simulink model "rotation_controllers_test"  (Simulink 8.8)
settings: Solver=ode4  StartTime=0.0  StopTime=10.0  FixedStep=1e-4  RelTol=1e-3  EnableMultiTasking=on
values from neighbouring files (symbols this model uses):
  g = [0;0;-9.81]    [rotation_controllers_test_start.m]
  I_B_C = inertiavector2matrix([4, 8, 15,-1,-2,-0.5])    [rotation_controllers_test_start.m]
  m = 1.5    [rotation_controllers_test_start.m]
libraries: lib_cartesian_controllers x2, rigid_body_dynamics x2, transformations_lib x2
settings Model: SuppressorTable=22 serialization::archive 11 0 3 0 0 0 11 0  Creator=schappler  LastModifiedBy=schappler
settings DataIOCC: LimitDataPoints=off  SaveFormat=StructureWithTime  SignalLoggingSaveFormat=Dataset
settings DebuggingCC: UnderspecifiedInitializationDetection=Simplified  MergeDetectMultiDrivingBlocksExec=error  FcnCallInpInsideContextMsg=error  StateNameClashWarn=none
settings GRTTargetCC: CombineOutputUpdateFcns=on  GRTInterface=off

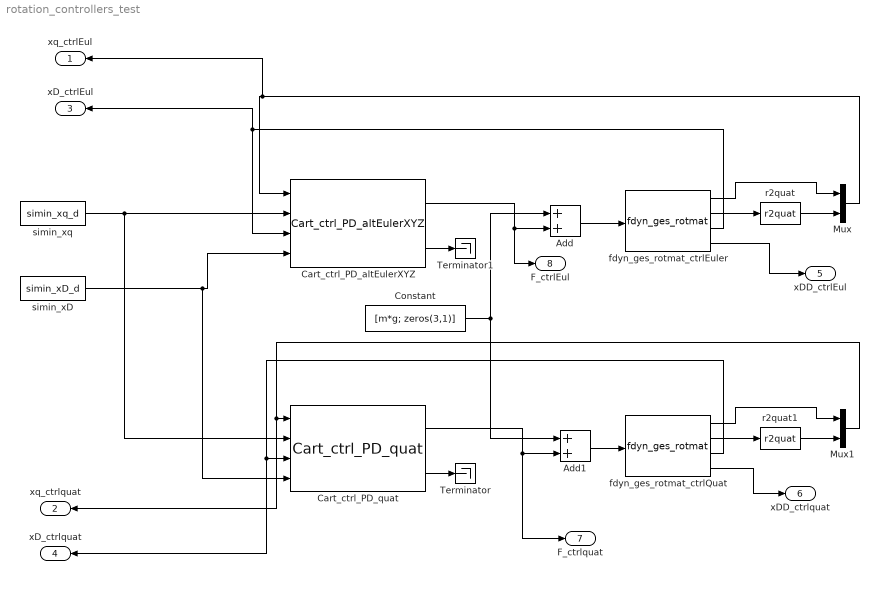
== system rotation_controllers_test ==
  Add : Sum
  Add1 : Sum
  Cart_ctrl_PD_altEulerXYZ : lib_cartesian_controllers/Cart_ctrl_PD_altEulerXYZ  k_P_p=k_P_p_C1  k_P_r=k_P_r_C1  k_D_p=k_D_p_C1  k_D_r=k_D_r_C1
  Cart_ctrl_PD_quat : lib_cartesian_controllers/Cart_ctrl_PD_quat  k_P_p=k_P_p_C2  k_P_r=k_P_r_C2  k_D_p=k_D_p_C2  k_D_r=k_D_r_C2
  Constant : Constant  Value=[m*g; zeros(3,1)]
  Mux : Mux  Inputs=[3 4]
  Mux1 : Mux  Inputs=[3 4]
  Terminator : Terminator
  Terminator1 : Terminator
  fdyn_ges_rotmat_ctrlEuler : rigid_body_dynamics/fdyn_ges_rotmat  I=I_B_C  m=m  r0=r0  rD0=rD0  R_t0=R_W_B_t0  omega0_t0=omega0_t0  r_B_B_C=r_B_B_C
  fdyn_ges_rotmat_ctrlQuat : rigid_body_dynamics/fdyn_ges_rotmat  I=I_B_C  m=m  r0=r0  rD0=rD0  R_t0=R_W_B_t0  omega0_t0=omega0_t0  r_B_B_C=r_B_B_C
  r2quat : transformations_lib/r2quat
  r2quat1 : transformations_lib/r2quat
  simin_xD : FromWorkspace  VariableName=simin_xD_d  SampleTime=0
  simin_xq : FromWorkspace  VariableName=simin_xq_d  SampleTime=0
  xq_ctrlEul : Outport
  xq_ctrlquat : Outport  Port=2
  xD_ctrlEul : Outport  Port=3
  xD_ctrlquat : Outport  Port=4
  xDD_ctrlEul : Outport  Port=5
  xDD_ctrlquat : Outport  Port=6
  F_ctrlquat : Outport  Port=7
  F_ctrlEul : Outport  Port=8
  wires:
  Cart_ctrl_PD_altEulerXYZ/1 -> Add/2, F_ctrlEul/1
  Cart_ctrl_PD_quat/1 -> Add1/2, F_ctrlquat/1
  fdyn_ges_rotmat_ctrlEuler/2 -> r2quat/1
  r2quat/1 -> Mux/2
  fdyn_ges_rotmat_ctrlEuler/1 -> Mux/1
  Mux/1 -> xq_ctrlEul/1, Cart_ctrl_PD_altEulerXYZ/1
  fdyn_ges_rotmat_ctrlEuler/3 -> xD_ctrlEul/1, Cart_ctrl_PD_altEulerXYZ/3
  fdyn_ges_rotmat_ctrlQuat/2 -> r2quat1/1
  r2quat1/1 -> Mux1/2
  fdyn_ges_rotmat_ctrlQuat/1 -> Mux1/1
  Mux1/1 -> xq_ctrlquat/1, Cart_ctrl_PD_quat/1
  fdyn_ges_rotmat_ctrlQuat/3 -> xD_ctrlquat/1, Cart_ctrl_PD_quat/3
  simin_xq/1 -> Cart_ctrl_PD_quat/2, Cart_ctrl_PD_altEulerXYZ/2
  simin_xD/1 -> Cart_ctrl_PD_quat/4, Cart_ctrl_PD_altEulerXYZ/4
  fdyn_ges_rotmat_ctrlEuler/4 -> xDD_ctrlEul/1
  fdyn_ges_rotmat_ctrlQuat/4 -> xDD_ctrlquat/1
  Add/1 -> fdyn_ges_rotmat_ctrlEuler/1
  Constant/1 -> Add/1, Add1/1
  Add1/1 -> fdyn_ges_rotmat_ctrlQuat/1
  Cart_ctrl_PD_quat/2 -> Terminator/1
  Cart_ctrl_PD_altEulerXYZ/2 -> Terminator1/1
